simulink model "roll_attitude_hold"  (Simulink 7.7)
settings: Solver=ode3  StartTime=0.0  StopTime=10.0  RelTol=1e-3
undefined symbols (not defined in the file): a_theta_1, a_theta_2, k_d_theta, k_p_theta
settings Model: Creator=prattmic  LastModifiedBy=prattmic
settings OptimizationCC: InlineParams=on
settings HardwareCC: ProdLargestAtomicInteger=Long  ProdLargestAtomicFloat=Double  ProdEndianess=LittleEndian  ProdHWDeviceType=ARM Compatible->ARM Cortex
settings RTWCC: GenCodeOnly=on

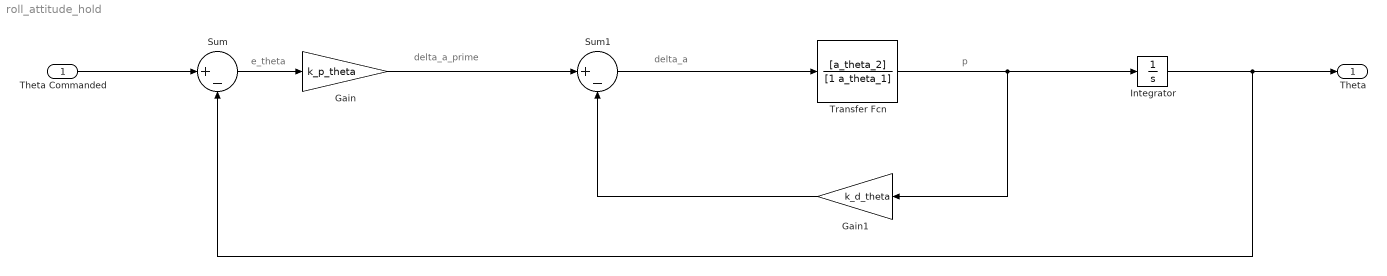
== system roll_attitude_hold ==
  note: p
  note: e_theta
  note: delta_a_prime
  note: delta_a
  Theta Commanded : Inport
  Gain : Gain  Gain=k_p_theta
  Gain1 : Gain  Gain=k_d_theta
  Integrator : Integrator
  Sum : Sum  Inputs=|+-
  Sum1 : Sum  Inputs=|+-
  Transfer Fcn : TransferFcn  Numerator=[a_theta_2]  Denominator=[1 a_theta_1]
  Theta : Outport
  wires:
  Integrator/1 -> Theta/1, Sum/2
  Transfer Fcn/1 -> Integrator/1, Gain1/1
  Theta Commanded/1 -> Sum/1
  Sum/1 -> Gain/1
  Gain/1 -> Sum1/1
  Sum1/1 -> Transfer Fcn/1
  Gain1/1 -> Sum1/2
